simulink library "MOTH"  (R2016b)
settings: Solver=ode45  StartTime=0.0  StopTime=10.0  RelTol=1e-3  EnableMultiTasking=on
undefined symbols (not defined in the file): CAL_backwardErrorVal, CAL_ErrorLowerLimit, CAL_ErrorUpperLimit, CAL_forwardStartIncr, CAL_MOTOR_HIGH, CAL_MOTOR_LOW, CONST_EndOfLineEnableFlg, CONST_NegOne, CONST_noVelocity, ENU_BACKWARD, ENU_FORWARD, ENU_STOP
libraries: simulink_need_slupdate x1
settings Model: Creator=oelkawok  LastModifiedBy=oelkawok
settings DataIOCC: LimitDataPoints=on
settings OptimizationCC: LifeSpan=inf
settings DebuggingCC: AllowSymbolicDim=off  SFUnexpectedBacktrackingDiag=warning  SFNoUnconditionalDefaultTransitionDiag=warning  SFExecutionAtInitializationDiag=none
settings GRTTargetCC: TargetLangStandard=C89/C90 (ANSI)  GeneratePreprocessorConditionals=Disable all
settings ConfigComp: CovMetricSettings=dw  CovHtmlReporting=on  CovSaveCumulativeToWorkspaceVar=on  CovSaveSingleToWorkspaceVar=on  CovExternalEMLEnable=off

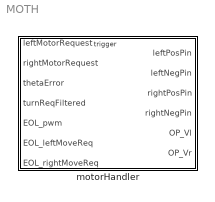
== system MOTH ==
  motorHandler : Subsystem

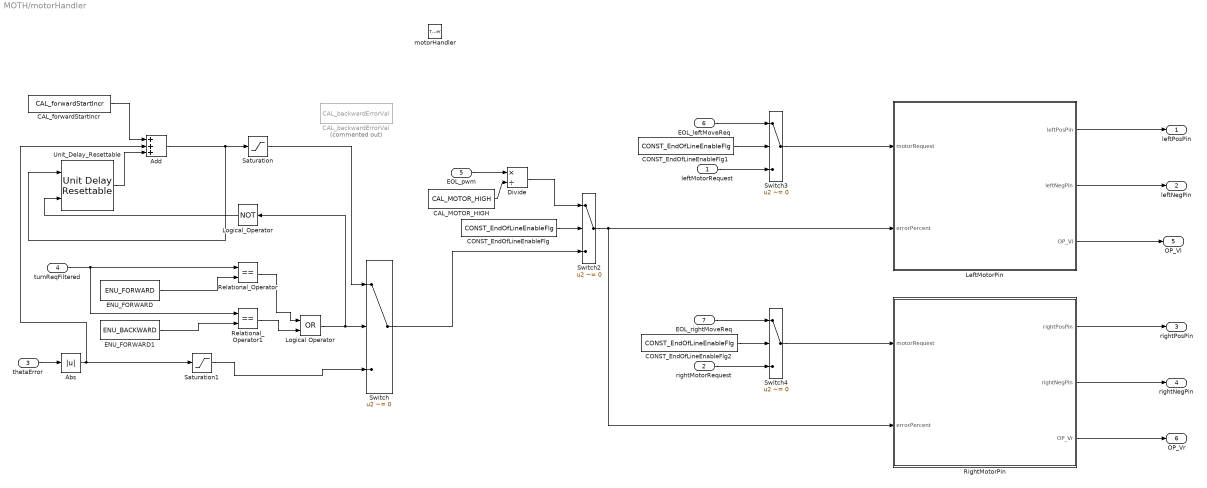
== system MOTH/motorHandler ==
  leftMotorRequest : Inport
  rightMotorRequest : Inport  Port=2
  thetaError : Inport  Port=3
  turnReqFiltered : Inport  Port=4
  EOL_pwm : Inport  Port=5
  EOL_leftMoveReq : Inport  Port=6
  EOL_rightMoveReq : Inport  Port=7
  motorHandler : TriggerPort  TriggerType=function-call  VariantControl=Variant
      settings: AttributesFormatString=Mode: %<StatesWhenEnabling>
  Abs : Abs
  Add : Sum  Inputs=+++
  CAL_MOTOR_HIGH : Constant  Value=CAL_MOTOR_HIGH
  CAL_backwardErrorVal : Constant  Commented=on  Value=CAL_backwardErrorVal
  CAL_forwardStartIncr : Constant  Value=CAL_forwardStartIncr
  CONST_EndOfLineEnableFlg : Constant  Value=CONST_EndOfLineEnableFlg
  CONST_EndOfLineEnableFlg1 : Constant  Value=CONST_EndOfLineEnableFlg
  CONST_EndOfLineEnableFlg2 : Constant  Value=CONST_EndOfLineEnableFlg
  Divide : Product  Inputs=*/
  ENU_FORWARD : Constant  Value=ENU_FORWARD
  ENU_FORWARD1 : Constant  Value=ENU_BACKWARD
  LeftMotorPin : Subsystem
  Logical Operator : Logic  Operator=OR  AllPortsSameDT=off  OutDataTypeStr=boolean
  Logical_Operator : Logic  Operator=NOT  AllPortsSameDT=off  OutDataTypeStr=boolean
  Relational_Operator : RelationalOperator  Operator===  OutDataTypeStr=boolean  RndMeth=Nearest
  Relational_Operator1 : RelationalOperator  Operator===  OutDataTypeStr=boolean  RndMeth=Nearest
  RightMotorPin : Subsystem
  Saturation : Saturate  UpperLimit=CAL_ErrorUpperLimit  LowerLimit=0
      settings: AttributesFormatString=|
      | upper = %<UpperLimit>
      | lower = %<LowerLimit>
  Saturation1 : Saturate  UpperLimit=CAL_ErrorUpperLimit  LowerLimit=CAL_ErrorLowerLimit
      settings: AttributesFormatString=|
      | upper = %<UpperLimit>
      | lower = %<LowerLimit>
  Switch{,2..4} (4 alike) : Switch  Criteria=u2 ~= 0
  Unit_Delay_Resettable : simulink_need_slupdate/Unit Delay Resettable  vinit=0.001  tsamp=-1
  leftPosPin : Outport
      settings: AttributesFormatString=|
      | Mode: %<OutputWhenDisabled>
      | Init: %<InitialOutput>
  leftNegPin : Outport  Port=2
      settings: AttributesFormatString=|
      | Mode: %<OutputWhenDisabled>
      | Init: %<InitialOutput>
  rightPosPin : Outport  Port=3
      settings: AttributesFormatString=|
      | Mode: %<OutputWhenDisabled>
      | Init: %<InitialOutput>
  rightNegPin : Outport  Port=4
      settings: AttributesFormatString=|
      | Mode: %<OutputWhenDisabled>
      | Init: %<InitialOutput>
  OP_Vl : Outport  Port=5
      settings: AttributesFormatString=|
      | Mode: %<OutputWhenDisabled>
      | Init: %<InitialOutput>
  OP_Vr : Outport  Port=6
      settings: AttributesFormatString=|
      | Mode: %<OutputWhenDisabled>
      | Init: %<InitialOutput>
  wires:
  Logical Operator/1 -> Switch/2, Logical_Operator/1
  Relational_Operator1/1 -> Logical Operator/2
  ENU_FORWARD1/1 -> Relational_Operator1/2
  Switch/1 -> Switch2/3
  Switch2/1 -> LeftMotorPin/2(errorPercent), RightMotorPin/2(errorPercent)
  Divide/1 -> Switch2/1
  CAL_MOTOR_HIGH/1 -> Divide/2
  EOL_pwm/1 -> Divide/1
  CONST_EndOfLineEnableFlg/1 -> Switch2/2
  RightMotorPin/3(OP_Vr) -> OP_Vr/1
  LeftMotorPin/3(OP_Vl) -> OP_Vl/1
  LeftMotorPin/1(leftPosPin) -> leftPosPin/1
  RightMotorPin/2(rightNegPin) -> rightNegPin/1
  thetaError/1 -> Abs/1
  turnReqFiltered/1 -> Relational_Operator/1, Relational_Operator1/1
  ENU_FORWARD/1 -> Relational_Operator/2
  Abs/1 -> Add/2, Saturation1/1
  Unit_Delay_Resettable/1 -> Add/3
  Add/1 -> Unit_Delay_Resettable/1, Saturation/1
  Saturation/1 -> Switch/1
  Relational_Operator/1 -> Logical Operator/1
  CAL_forwardStartIncr/1 -> Add/1
  Logical_Operator/1 -> Unit_Delay_Resettable/2
  Saturation1/1 -> Switch/3
  leftMotorRequest/1 -> Switch3/3
  CONST_EndOfLineEnableFlg1/1 -> Switch3/2
  EOL_leftMoveReq/1 -> Switch3/1
  Switch3/1 -> LeftMotorPin/1(motorRequest)
  EOL_rightMoveReq/1 -> Switch4/1
  CONST_EndOfLineEnableFlg2/1 -> Switch4/2
  rightMotorRequest/1 -> Switch4/3
  Switch4/1 -> RightMotorPin/1(motorRequest)
  RightMotorPin/1(rightPosPin) -> rightPosPin/1
  LeftMotorPin/2(leftNegPin) -> leftNegPin/1

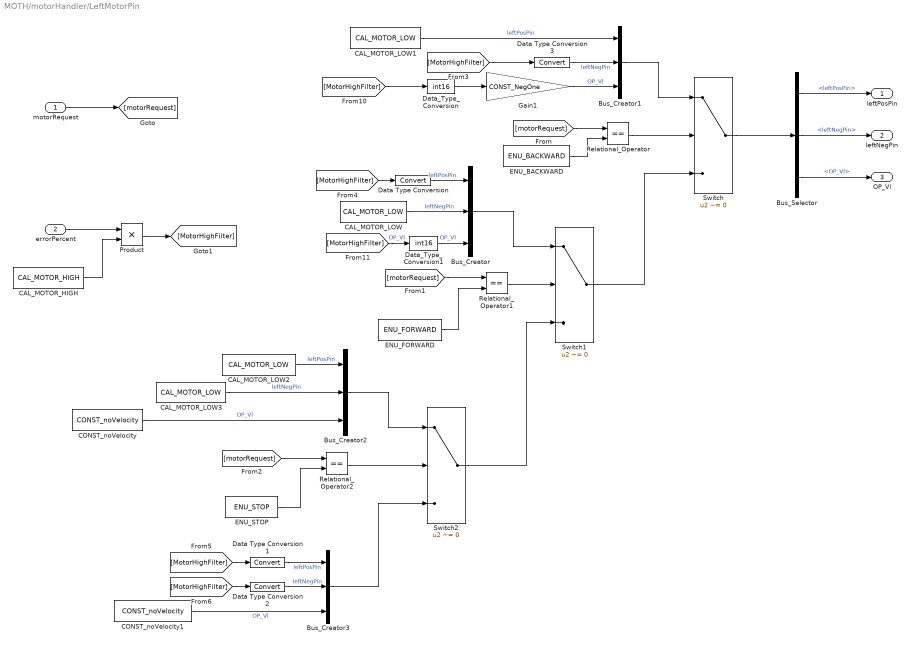
== system MOTH/motorHandler/LeftMotorPin ==
  motorRequest : Inport
  errorPercent : Inport  Port=2
  Bus_Creator{,1..3} (4 alike) : BusCreator  Inputs=3
  Bus_Selector : BusSelector  OutputSignals=leftPosPin,leftNegPin,OP_Vl
  CAL_MOTOR_HIGH : Constant  Value=CAL_MOTOR_HIGH
  CAL_MOTOR_LOW{,1..3} (4 alike) : Constant  Value=CAL_MOTOR_LOW
  CONST_noVelocity : Constant  Value=CONST_noVelocity
  CONST_noVelocity1 : Constant  Value=CONST_noVelocity
  Data Type Conversion{,1..3} (4 alike) : DataTypeConversion
  Data_Type_Conversion : DataTypeConversion  OutDataTypeStr=int16
  Data_Type_Conversion1 : DataTypeConversion  OutDataTypeStr=int16
  ENU_BACKWARD : Constant  Value=ENU_BACKWARD
  ENU_FORWARD : Constant  Value=ENU_FORWARD
  ENU_STOP : Constant  Value=ENU_STOP
  Gain1 : Gain  Gain=CONST_NegOne  OutDataTypeStr=int16
  Product : Product  OutDataTypeStr=uint8
  Relational_Operator : RelationalOperator  Operator===  OutDataTypeStr=boolean  RndMeth=Nearest
  Relational_Operator1 : RelationalOperator  Operator===  OutDataTypeStr=boolean  RndMeth=Nearest
  Relational_Operator2 : RelationalOperator  Operator===  OutDataTypeStr=boolean  RndMeth=Nearest
  Switch : Switch  Criteria=u2 ~= 0
  Switch1 : Switch  Criteria=u2 ~= 0
  Switch2 : Switch  Criteria=u2 ~= 0
  leftPosPin : Outport
  leftNegPin : Outport  Port=2
  OP_Vl : Outport  Port=3
  wires:
  Bus_Selector/3 -> OP_Vl/1  "<OP_Vl>"
  Bus_Selector/2 -> leftNegPin/1  "<leftNegPin>"
  Bus_Selector/1 -> leftPosPin/1  "<leftPosPin>"
  Data Type Conversion3/1 -> Bus_Creator1/2  "leftNegPin"
  Data Type Conversion2/1 -> Bus_Creator3/2  "leftNegPin"
  Data Type Conversion1/1 -> Bus_Creator3/1  "leftPosPin"
  Data Type Conversion/1 -> Bus_Creator/1  "leftPosPin"
  Product/1 -> [MotorHighFilter]
  CAL_MOTOR_HIGH/1 -> Product/2
  errorPercent/1 -> Product/1
  Relational_Operator1/1 -> Switch1/2
  CAL_MOTOR_LOW/1 -> Bus_Creator/2  "leftNegPin"
  [MotorHighFilter] -> Data Type Conversion/1
  [MotorHighFilter] -> Data Type Conversion3/1
  ENU_BACKWARD/1 -> Relational_Operator/2
  Relational_Operator/1 -> Switch/2
  ENU_FORWARD/1 -> Relational_Operator1/2
  ENU_STOP/1 -> Relational_Operator2/2
  CAL_MOTOR_LOW1/1 -> Bus_Creator1/1  "leftPosPin"
  Switch1/1 -> Switch/3
  CAL_MOTOR_LOW2/1 -> Bus_Creator2/1  "leftPosPin"
  Bus_Creator/1 -> Switch1/1
  Bus_Creator2/1 -> Switch2/1
  Bus_Creator1/1 -> Switch/1
  [motorRequest] -> Relational_Operator2/1
  [MotorHighFilter] -> Data Type Conversion2/1
  Relational_Operator2/1 -> Switch2/2
  CAL_MOTOR_LOW3/1 -> Bus_Creator2/2  "leftNegPin"
  [MotorHighFilter] -> Data Type Conversion1/1
  Switch2/1 -> Switch1/3
  Bus_Creator3/1 -> Switch2/3
  motorRequest/1 -> [motorRequest]
  [motorRequest] -> Relational_Operator/1
  [motorRequest] -> Relational_Operator1/1
  Switch/1 -> Bus_Selector/1
  [MotorHighFilter] -> Data_Type_Conversion/1
  Gain1/1 -> Bus_Creator1/3  "OP_Vl"
  [MotorHighFilter] -> Data_Type_Conversion1/1  "OP_Vl"
  CONST_noVelocity/1 -> Bus_Creator2/3  "OP_Vl"
  CONST_noVelocity1/1 -> Bus_Creator3/3  "OP_Vl"
  Data_Type_Conversion/1 -> Gain1/1
  Data_Type_Conversion1/1 -> Bus_Creator/3  "OP_Vl"

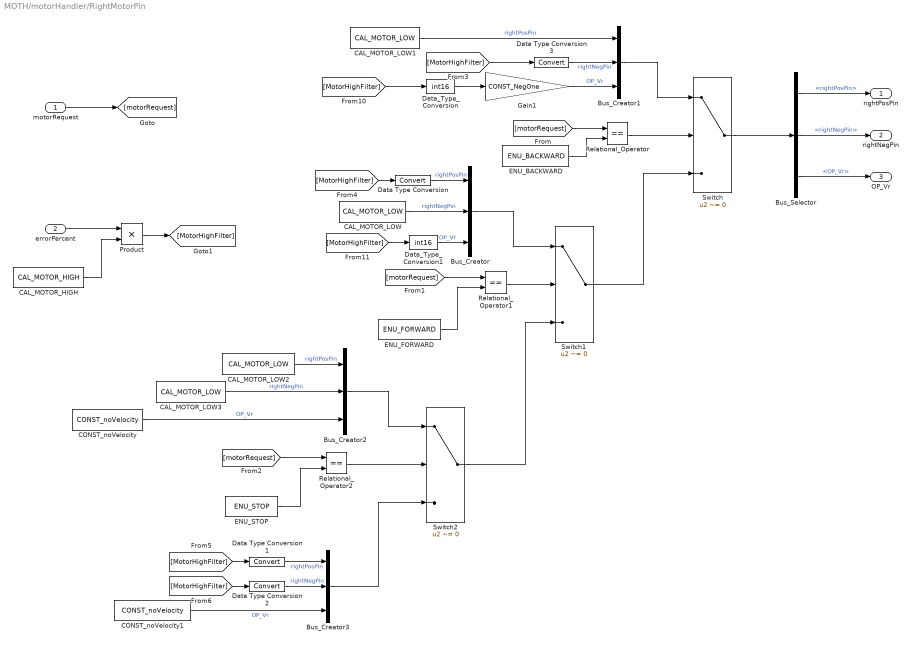
== system MOTH/motorHandler/RightMotorPin ==
  motorRequest : Inport
  errorPercent : Inport  Port=2
  Bus_Creator{,1..3} (4 alike) : BusCreator  Inputs=3
  Bus_Selector : BusSelector  OutputSignals=rightPosPin,rightNegPin,OP_Vr
  CAL_MOTOR_HIGH : Constant  Value=CAL_MOTOR_HIGH
  CAL_MOTOR_LOW{,1..3} (4 alike) : Constant  Value=CAL_MOTOR_LOW
  CONST_noVelocity : Constant  Value=CONST_noVelocity
  CONST_noVelocity1 : Constant  Value=CONST_noVelocity
  Data Type Conversion{,1..3} (4 alike) : DataTypeConversion
  Data_Type_Conversion : DataTypeConversion  OutDataTypeStr=int16
  Data_Type_Conversion1 : DataTypeConversion  OutDataTypeStr=int16
  ENU_BACKWARD : Constant  Value=ENU_BACKWARD
  ENU_FORWARD : Constant  Value=ENU_FORWARD
  ENU_STOP : Constant  Value=ENU_STOP
  Gain1 : Gain  Gain=CONST_NegOne  OutDataTypeStr=int16
  Product : Product  OutDataTypeStr=uint8
  Relational_Operator : RelationalOperator  Operator===  OutDataTypeStr=boolean  RndMeth=Nearest
  Relational_Operator1 : RelationalOperator  Operator===  OutDataTypeStr=boolean  RndMeth=Nearest
  Relational_Operator2 : RelationalOperator  Operator===  OutDataTypeStr=boolean  RndMeth=Nearest
  Switch : Switch  Criteria=u2 ~= 0
  Switch1 : Switch  Criteria=u2 ~= 0
  Switch2 : Switch  Criteria=u2 ~= 0
  rightPosPin : Outport
  rightNegPin : Outport  Port=2
  OP_Vr : Outport  Port=3
  wires:
  Data_Type_Conversion1/1 -> Bus_Creator/3  "OP_Vr"
  Data_Type_Conversion/1 -> Gain1/1
  CONST_noVelocity1/1 -> Bus_Creator3/3  "OP_Vr"
  CONST_noVelocity/1 -> Bus_Creator2/3  "OP_Vr"
  [MotorHighFilter] -> Data_Type_Conversion1/1
  Gain1/1 -> Bus_Creator1/3  "OP_Vr"
  [MotorHighFilter] -> Data_Type_Conversion/1
  Switch/1 -> Bus_Selector/1
  [motorRequest] -> Relational_Operator1/1
  [motorRequest] -> Relational_Operator/1
  motorRequest/1 -> [motorRequest]
  Bus_Creator3/1 -> Switch2/3
  Switch2/1 -> Switch1/3
  [MotorHighFilter] -> Data Type Conversion1/1
  CAL_MOTOR_LOW3/1 -> Bus_Creator2/2  "rightNegPin"
  Relational_Operator2/1 -> Switch2/2
  [MotorHighFilter] -> Data Type Conversion2/1
  [motorRequest] -> Relational_Operator2/1
  Bus_Creator1/1 -> Switch/1
  Bus_Creator2/1 -> Switch2/1
  Bus_Creator/1 -> Switch1/1
  CAL_MOTOR_LOW2/1 -> Bus_Creator2/1  "rightPosPin"
  Switch1/1 -> Switch/3
  CAL_MOTOR_LOW1/1 -> Bus_Creator1/1  "rightPosPin"
  ENU_STOP/1 -> Relational_Operator2/2
  ENU_FORWARD/1 -> Relational_Operator1/2
  Relational_Operator/1 -> Switch/2
  ENU_BACKWARD/1 -> Relational_Operator/2
  [MotorHighFilter] -> Data Type Conversion3/1
  [MotorHighFilter] -> Data Type Conversion/1
  CAL_MOTOR_LOW/1 -> Bus_Creator/2  "rightNegPin"
  Relational_Operator1/1 -> Switch1/2
  errorPercent/1 -> Product/1
  CAL_MOTOR_HIGH/1 -> Product/2
  Product/1 -> [MotorHighFilter]
  Data Type Conversion/1 -> Bus_Creator/1  "rightPosPin"
  Data Type Conversion1/1 -> Bus_Creator3/1  "rightPosPin"
  Data Type Conversion2/1 -> Bus_Creator3/2  "rightNegPin"
  Data Type Conversion3/1 -> Bus_Creator1/2  "rightNegPin"
  Bus_Selector/1 -> rightPosPin/1  "<rightPosPin>"
  Bus_Selector/2 -> rightNegPin/1  "<rightNegPin>"
  Bus_Selector/3 -> OP_Vr/1  "<OP_Vr>"
